simulink model "unitree_a1_bounding"  (R2022b)
settings: Solver=VariableStepAuto  StartTime=0.0  StopTime=10.0  RelTol=1e-3
values from neighbouring files (symbols this model uses):
  m = 12    [mpc.m]    (also in mpc_soln.m; qp_soln.m)
  N = 50    [mpc.m]    (also in mpc_caller.m = params.N; qp_caller.m = params.N)
  X = [p; reshape(R, [9 1]); v; R'*w]    [mpc_caller.m]    (also in qp_caller.m)
undefined symbols (not defined in the file or in its folder): Y, Z
libraries: sm_lib x214, nesl_utility x117, simulink x3
(part 5 of 5)

== matlab function unitree_a1_bounding/Subsystem13/MATLAB Function1 ==
  data: p input; v input; w input; tau output; R input; q input; vd input; wd input; p1 input; p2 input; p3 input; p4 input; t input; F output; task input
function [tau, F] = mpc_controller_wrapper(p, v, w, R, q, vd, wd, p1, p2, p3, p4, t, task)
    [tau, F] = mpc_caller(p, v, w, R, q, vd, wd, p1, p2, p3, p4, t, task);
end

== matlab function unitree_a1_bounding/MATLAB Function ==
  data: q input; tau output; q_dot input; qd input; qd_dot input
function tau = pd_controller(q, q_dot, qd, qd_dot)
    Kp = 1e3; Kd = 1e3;
    
    tau = Kp * (qd - q) + Kd * (qd_dot - q_dot);

== matlab function unitree_a1_bounding/MATLAB Function1 ==
  data: tau_pd input; tau output; tau_mpc input; tau_swing input; tau_qp input; q input; q_dot input; qd input; qd_dot input; t input
function tau = choose_controller(tau_pd, tau_mpc, tau_swing, tau_qp, q, q_dot, qd, qd_dot, t)

select_leg = [0;0;1;0];

if t >= get_gait_params().t_start
    tau = tau_mpc + tau_swing;
%     tau = tau_mpc + tau_swing.*[select_leg;select_leg;select_leg;];
    %tau = tau_pd.*[1-select_leg; 1-select_leg; 1-select_leg] + tau_swing.*[select_leg; select_leg; select_leg];
    %tau = tau_qp.*[1-select_leg; 1-select_leg; 1-select_leg] + tau_swing.*[select_leg; select_leg; select_leg];

else
    tau = tau_pd;
%     csvwrite("taupd.csv", tau_pd);
    for i=1:12
        fprintf("%f %f\n", i, tau(i));
    end
end

== matlab function unitree_a1_bounding/MATLAB Function2 ==
  data: p input; R input; tau output; v input; p_hip input; p_foot input; v_foot input; q input; vd input; w input; t input; pd_foot output; vd_foot output; pfinal_foot output; Fswing output; task input; theta output double
function [tau, pd_foot, vd_foot, pfinal_foot, Fswing, theta] = swing_controller(p, R, v, p_hip, p_foot, v_foot, q, vd, w, t, task)

pfinal_foot = zeros(12,1);
theta = 0;

if task == 0 % standing
    [tau, pd_foot, vd_foot, Fswing] = foot_placement_standing(p, R, v, p_hip, p_foot, v_foot, q, t);
elseif task == 1 % walking
    [tau, pd_foot, vd_foot, pfinal_foot, Fswing] = foot_placement_walking(p, R, v, p_hip, p_foot, v_foot, q, vd, t);
elseif task == 2 % turning
    [tau, pd_foot, vd_foot, pfinal_foot, Fswing] = foot_placement_turning(p, R, v, p_hip, p_foot, v_foot, q, vd, w, t);
elseif  task == 3 % running
    %[tau, pd_foot, vd_foot, pfinal_foot, Fswing] = foot_placement_running(p, R, v, p_hip, p_foot, v_foot, q, vd, t);
    [tau, pd_foot, vd_foot, pfinal_foot, Fswing] = foot_placement_bounding(p, R, v, p_hip, p_foot, v_foot, q, vd, t);
else  
    [tau, pd_foot, vd_foot, Fswing] = foot_placement_standing(p, R, v, p_hip, p_foot, v_foot, q, t);
end


% select_leg = [0;0;1;0];
% tau = tau.*[select_leg;select_leg;select_leg;]

== matlab function unitree_a1_bounding/MATLAB Function3 ==
  data: p input; v input; w input; tau output; R input; q input; p1 input; p2 input; p3 input; p4 input; t input; F output
function [tau, F] = qp_controller_wrapper(p, v, w, R, q, p1, p2, p3, p4, t)
    [tau, F] = qp_caller(p, v, w, R, q, p1, p2, p3, p4, t);
end
